simulink model "clearing_faulted_segment_travelling_Wave"  (R2018a)
settings: Solver=ode23t  StartTime=0.0  StopTime=2  MaxStep=1e-3  RelTol=1e-3
values from neighbouring files (symbols this model uses):
  AC_lim = [1.5 -1.5]    [MT_HVDC_initialize.m]
  C_pm = 10.48e-3    (= 0.01048)    [MT_HVDC_initialize.m]
  ccsc_lim = [1.0 -1.0]    [MT_HVDC_initialize.m]
  DC_lim = [1.05 -1.05]    [MT_HVDC_initialize.m]
  f = 50    [MT_HVDC_initialize.m]
  Fc = 50    [MT_HVDC_initialize.m]
  Fn_filter = 1000    [MT_HVDC_initialize.m]
  Ireg_lim_i = [1.5, -1.5]    [MT_HVDC_initialize.m]
  Ireg_lim_r = [1.5, -1.5]    [MT_HVDC_initialize.m]
  Ki_ACreg_i = 260    [MT_HVDC_initialize.m]
  Ki_ccsc = 5    [MT_HVDC_initialize.m]
  Ki_DCreg_r = 150    [MT_HVDC_initialize.m]
  Ki_Ireg_i = 200    [MT_HVDC_initialize.m]
  Ki_Ireg_r = 100    [MT_HVDC_initialize.m]
  Ki_R_inv = 150000    [MT_HVDC_initialize.m]
  Ki_R_rec = 5000    [MT_HVDC_initialize.m]
  Kp_ACreg_i = 2    [MT_HVDC_initialize.m]
  Kp_ccsc = 1    [MT_HVDC_initialize.m]
  Kp_DCreg_r = 8    [MT_HVDC_initialize.m]
  Kp_Ireg_i = 2    [MT_HVDC_initialize.m]
  Kp_Ireg_r = 2    [MT_HVDC_initialize.m]
  Kp_R_inv = 0.001    [MT_HVDC_initialize.m]
  Kp_R_rec = 0.001    [MT_HVDC_initialize.m]
  L1_pu = 0.109    [MT_HVDC_initialize.m]
  L2_pu = 0.0824    [MT_HVDC_initialize.m]
  L_arm = L_arm_pu*Z_base66/w    [MT_HVDC_initialize.m]
  L_arm_pu = 0.15    [MT_HVDC_initialize.m]
  L_int = X_int/w    [MT_HVDC_initialize.m]
  n = 50    [MT_HVDC_initialize.m]
  n2 = 50    [MT_HVDC_initialize.m]
  P_nom = 220e6    (= 220000000)    [MT_HVDC_initialize.m]
  R1_pu = 0.00206    [MT_HVDC_initialize.m]
  R2_pu = 0.00206    [MT_HVDC_initialize.m]
  R_arm = 0.03    [MT_HVDC_initialize.m]
  R_arm_pu = R_arm/Z_base66    [MT_HVDC_initialize.m]
  R_int = sqrt((z_int_400^2)/(1+xr_ratio^2))    [MT_HVDC_initialize.m]
  Rg_T1 = 40    [MT_HVDC_initialize.m]
  S1_nom = P_nom    (= 220000000)    [MT_HVDC_initialize.m]
  S2_nom = P_nom    (= 220000000)    [MT_HVDC_initialize.m]
  T_fault = 1.4    [MT_HVDC_initialize.m]
  Ts_Control = 40e-6    (= 4e-05)    [MT_HVDC_initialize.m]
  Ts_Power = 20e-6    (= 2e-05)    [MT_HVDC_initialize.m]
  V1_prim = V_prim    (= 400000)    [MT_HVDC_initialize.m]
  V1_sec = V_grid    (= 66000)    [MT_HVDC_initialize.m]
  V2_prim = V_grid    (= 66000)    [MT_HVDC_initialize.m]
  V2_sec = 18e3    (= 18000)    [MT_HVDC_initialize.m]
  V_ac_ref = 1.035    [MT_HVDC_initialize.m]
  V_grid = 66e3    (= 66000)    [MT_HVDC_initialize.m]
  V_prim = 400e3    (= 400000)    [MT_HVDC_initialize.m]
  Vc_pm_r = 0*Vdc_nom/n    (= 0)    [MT_HVDC_initialize.m]
  Vdc_nom = 135e3    (= 135000)    [MT_HVDC_initialize.m]
  w = 2*pi*f    (= 314.159265359)    [MT_HVDC_initialize.m]
  z0z1 = 0.8    [MT_HVDC_initialize.m]
  Zeta_filter = 1    [MT_HVDC_initialize.m]
undefined symbols (not defined in the file or in its folder): D1, Delta, DiscIntNeverNeededParam
libraries: powerlib x417, powerlib_meascontrol x130, simulink x84, powerlib_extras x8, simulink_extras x5
(part 7 of 17)

== system clearing_faulted_segment_travelling_Wave/Startup Simulation - Guide ==
  note: Startup guide:
      | 1. Set inititial submodule capacitor voltages to zero in script
      | ********************Sequencer in following order**********************
      | 2. Set time for energize grid filter/transformers T_energize (0.1s)
      | 3. Set time for Circulating Current Suppression T_circ (0.1s)
      | 4. Set time for converter energization T_startup (0.4s)
      | 5. Set time for DC Regulator T_DC_Reg (0.4s)
      | 6. Set time for AC RMS Regulator T_AC_Reg (0.7s)
      | 7. Set time for load switching T_Load_nom (1.0s)

== system clearing_faulted_segment_travelling_Wave/Subsystem ==
  DC regulator TURN ON - (id reference for rectifier) : Step  Time=0.2  SampleTime=0
  Enable AC RMS regulator TURN ON - (id reference for inverter) : Step  Time=0.3  SampleTime=0
  Enable Circulating Current Suppresion : Step  Time=0.1  SampleTime=0
  Switch on load network : Step  Time=0.4  SampleTime=0
  tag scope: T_AC_Reg=global, T_DC_Reg=global, T_Load_nom=global, T_circ_i=global, T_circ_r=global
  wires:
  DC regulator TURN ON - (id reference for rectifier)/1 -> [T_DC_Reg]
  Enable Circulating Current Suppresion/1 -> [T_circ_i], [T_circ_r]
  Enable AC RMS regulator TURN ON - (id reference for inverter)/1 -> [T_AC_Reg]
  Switch on load network/1 -> [T_Load_nom]

== system clearing_faulted_segment_travelling_Wave/Thyristor Static AC BREAKER - Active bypass system ==
  note: This thyristor bypass switch is used for investigation of fault current supply when a fault in the load network occurs, allowing selectivity of the network since the MMC inverter cannot supply this current without taking damage.
  note: To Use: Block inverter and rectifier with logic signal, and enable the thyristor bypass. A control logic might be implemented that automatically detects situation where bypass is needed.
  note: Thyristor Pulse Generation based on PLL syncronization from GRID
  note: Thyristor Bypass System;
      |  Two sync: grid and load
      |    Is the blocking done in both converter at the same time, or rectifier and then inverter?
  Block : Inport
  wt : Inport  Port=2
  Constant : Constant  Value=0
  Constant1 : Constant  Value=pi
  Current Measurement : powerlib/Measurements/Current Measurement  PhasorSimulation=off  OutputType=Complex  PSBequivalent=0
      settings: SourceProductName=Simscape Electrical
  Demux1 : Demux  Outputs=6
  Less Than : RelationalOperator  Operator=<  OutDataTypeStr=boolean  RndMeth=Simplest
  Less Than1 : RelationalOperator  Operator=<  OutDataTypeStr=boolean  RndMeth=Simplest
  Less Than2 : RelationalOperator  Operator=<  OutDataTypeStr=boolean  RndMeth=Simplest
  Logical Operator : Logic  Operator=NOT  AllPortsSameDT=off  OutDataTypeStr=boolean
  Logical Operator1 : Logic  Operator=NOT  AllPortsSameDT=off  OutDataTypeStr=boolean
  Logical Operator2 : Logic  Operator=NOT  AllPortsSameDT=off  OutDataTypeStr=boolean
  Mux : Mux  Inputs=6
  Scope : Scope  NumInputPorts=2
  Switch1 : Switch  Criteria=u2 > Threshold
  Terminator{,1..5} (6 alike) : Terminator
  Thyristor{,1..5} (6 alike) : powerlib/Power Electronics/Thyristor  Ron=0.001  Lon=0  Vf=0.8  IC=0  Rs=500  Cs=250e-9  Measurements=on
      settings: SourceProductName=Simscape Electrical
  Transport Delay : TransportDelay  DelayTime=(1/3)*(1/50)
  Transport Delay1 : TransportDelay  DelayTime=(2/3)*(1/50)
  Voltage Measurement : powerlib/Measurements/Voltage Measurement  PhasorSimulation=off  OutputType=Complex  PSBequivalent=0
      settings: SourceProductName=Simscape Electrical
  a : PMIOPort  Tag=PMCPort  Side=Left
  b : PMIOPort  Tag=PMCPort  Port=2  Side=Left
  c : PMIOPort  Tag=PMCPort  Port=3  Side=Left
  A : PMIOPort  Tag=PMCPort  Port=4  Side=Right
  " B" : PMIOPort  Tag=PMCPort  Port=5  Side=Right
  C : PMIOPort  Tag=PMCPort  Port=6  Side=Right
  wires:
  Block/1 -> Switch1/2
  Voltage Measurement/1 -> Scope/1
  Current Measurement/1 -> Scope/2
  Switch1/1 -> Demux1/1
  Constant/1 -> Switch1/1
  Constant1/1 -> Less Than/2, Less Than1/2, Less Than2/2
  Transport Delay/1 -> Less Than1/1
  Transport Delay1/1 -> Less Than2/1
  Less Than/1 -> Logical Operator/1, Mux/1
  wt/1 -> Transport Delay/1, Transport Delay1/1, Less Than/1
  Logical Operator/1 -> Mux/2
  Logical Operator1/1 -> Mux/4
  Logical Operator2/1 -> Mux/6
  Less Than1/1 -> Logical Operator1/1, Mux/3
  Less Than2/1 -> Logical Operator2/1, Mux/5
  Mux/1 -> Switch1/3
  Demux1/1 -> Thyristor/1
  Demux1/2 -> Thyristor1/1
  Demux1/3 -> Thyristor2/1
  Demux1/4 -> Thyristor3/1
  Demux1/5 -> Thyristor4/1
  Demux1/6 -> Thyristor5/1
  Thyristor/1 -> Terminator/1
  Thyristor2/1 -> Terminator1/1
  Thyristor5/1 -> Terminator2/1
  Thyristor1/1 -> Terminator4/1
  Thyristor3/1 -> Terminator3/1
  Thyristor4/1 -> Terminator5/1
  connections:
  Thyristor1/LConn1 -- Voltage Measurement/LConn2 -- Current Measurement/LConn1 -- Thyristor/RConn1
  Thyristor1/RConn1 -- Thyristor/LConn1 -- Voltage Measurement/LConn1 -- a/RConn1
  b/RConn1 -- Thyristor2/LConn1 -- Thyristor3/RConn1
  Thyristor3/LConn1 -- " B"/RConn1 -- Thyristor2/RConn1
  Thyristor4/LConn1 -- c/RConn1 -- Thyristor5/RConn1
  Thyristor4/RConn1 -- C/RConn1 -- Thyristor5/LConn1
  Current Measurement/RConn1 -- A/RConn1

== system clearing_faulted_segment_travelling_Wave/Controlsystem for Inverter/Dq0 Control ==
  I_ph : Inport
  V_ph : Inport  Port=2
  Circulating current suppression1 : Subsystem  VariantControl=Variant1
  Constant18 : Constant  Value=V_ac_ref
  Constant2 : Constant  Value=1/(Vdc_nom/2*sqrt(3)/sqrt(2)/V_grid)
  Goto8 : Goto  Commented=on  GotoTag=V_diffi_i  TagVisibility=global
  Inncer current loop - Positive and Negative Sequence Control : Subsystem
  "Measurement - dq0 positiveand negative sequence, - and zero sequence in alphabetta - Rectifier" : Subsystem
  Outer loop - AC RMS controller1 : Subsystem
  PWM Signal Generator - Inverter1 : Subsystem
  Rate Transition1 : RateTransition  OutPortSampleTime=Ts_Power
  Reactive power Set-point : Subsystem
  Zero Sequence Controller : Subsystem
  Control Signal1 : Outport
  tag scope: m_i_pn=global
  wires:
  "Measurement - dq0 positiveand negative sequence, - and zero sequence in alphabetta - Rectifier"/3(wt) -> Inncer current loop - Positive and Negative Sequence Control/5(wt)
  [T_AC_Reg] -> Outer loop - AC RMS controller1/3(Enable)
  [T_iq_reg_i] -> Reactive power Set-point/Enable, Reactive power Set-point/1(T_Qreg_on)
  [PQ_i] -> Reactive power Set-point/2(Q_ref)
  [I_arm_i] -> Circulating current suppression1/2(I_arm)
  [T_zero] -> Zero Sequence Controller/Enable, Zero Sequence Controller/3(Enable)
  [T_Block_i] -> PWM Signal Generator - Inverter1/2(Block)
  Zero Sequence Controller/1(V_zero_ref) -> Inncer current loop - Positive and Negative Sequence Control/7(V_ref_zero)
  Constant2/1 -> Inncer current loop - Positive and Negative Sequence Control/6(Vdc_pu)
  Inncer current loop - Positive and Negative Sequence Control/1(m_ref) -> [m_i_pn], Rate Transition1/1
  "Measurement - dq0 positiveand negative sequence, - and zero sequence in alphabetta - Rectifier"/4(V_zero) -> Zero Sequence Controller/1(V0_meas)
  PWM Signal Generator - Inverter1/1(g) -> Control Signal1/1
  Circulating current suppression1/1(V_diffi) -> Inncer current loop - Positive and Negative Sequence Control/8(V_diffi), Goto8/1
  Rate Transition1/1 -> PWM Signal Generator - Inverter1/1(U_ref)
  [T_circ_i] -> Circulating current suppression1/Enable, Circulating current suppression1/1(Enable)
  "Measurement - dq0 positiveand negative sequence, - and zero sequence in alphabetta - Rectifier"/5(I_zero) -> Zero Sequence Controller/2(I0_meas)
  Constant18/1 -> Outer loop - AC RMS controller1/1(Vac_ref)
  Outer loop - AC RMS controller1/1(Id_ref) -> Inncer current loop - Positive and Negative Sequence Control/1(id_pos_ref)
  Reactive power Set-point/1(Iq_ref) -> Inncer current loop - Positive and Negative Sequence Control/2(iq_pos_ref)
  "Measurement - dq0 positiveand negative sequence, - and zero sequence in alphabetta - Rectifier"/2(Vdq) -> Reactive power Set-point/3(Vdq+), Outer loop - AC RMS controller1/2(vdq+), Inncer current loop - Positive and Negative Sequence Control/4(Vdq+)
  "Measurement - dq0 positiveand negative sequence, - and zero sequence in alphabetta - Rectifier"/1(Idq) -> Inncer current loop - Positive and Negative Sequence Control/3(Idq+)
  I_ph/1 -> "Measurement - dq0 positiveand negative sequence, - and zero sequence in alphabetta - Rectifier"/2(I_ph)
  V_ph/1 -> "Measurement - dq0 positiveand negative sequence, - and zero sequence in alphabetta - Rectifier"/1(V_ph)

== system clearing_faulted_segment_travelling_Wave/Controlsystem for Inverter/Dq0 control with Dual Synchronous Reference Frame (DSRF) ==
  I_ph : Inport
  V_ph : Inport  Port=2
  Circulating current suppression1 : Subsystem  VariantControl=Variant1
  Constant : Constant  Value=V_ac_ref
  Constant2 : Constant  Value=1/(Vdc_nom/2*sqrt(3)/sqrt(2)/V_grid)
  Goto8 : Goto  Commented=on  GotoTag=V_diffi_i  TagVisibility=global
  Inncer current loop - Positive and Negative Sequence Control : Subsystem
  "Measurement - dq0 positiveand negative sequence, - and zero sequence in alphabetta2" : Subsystem
  Outer loop - AC RMS controller1 : Subsystem
  PWM Signal Generator - Inverter1 : Subsystem
  Rate Transition1 : RateTransition  OutPortSampleTime=Ts_Power
  Reactive power Set-point : Subsystem
  Zero Sequence Controller2 : Subsystem
  Control Signal1 : Outport
  tag scope: m_i_pn=global
  wires:
  "Measurement - dq0 positiveand negative sequence, - and zero sequence in alphabetta2"/3(Vdq+) -> Outer loop - AC RMS controller1/2(vdq+), Inncer current loop - Positive and Negative Sequence Control/5(Vdq+), Reactive power Set-point/3(Vdq+)
  "Measurement - dq0 positiveand negative sequence, - and zero sequence in alphabetta2"/4(Vdq-) -> Inncer current loop - Positive and Negative Sequence Control/6(Vdq-)
  [T_AC_Reg] -> Outer loop - AC RMS controller1/3(Enable)
  [T_iq_reg_i] -> Reactive power Set-point/Enable, Reactive power Set-point/1(T_Qreg_on)
  V_ph/1 -> "Measurement - dq0 positiveand negative sequence, - and zero sequence in alphabetta2"/2(V_ph)
  [PQ_i] -> Reactive power Set-point/2(Q_ref)
  I_ph/1 -> "Measurement - dq0 positiveand negative sequence, - and zero sequence in alphabetta2"/1(I_ph)
  Reactive power Set-point/1(Iq_ref) -> Inncer current loop - Positive and Negative Sequence Control/2(iq_pos_ref)
  "Measurement - dq0 positiveand negative sequence, - and zero sequence in alphabetta2"/2(Idq-) -> Inncer current loop - Positive and Negative Sequence Control/4(Idq-)
  [I_arm_i] -> Circulating current suppression1/2(I_arm)
  "Measurement - dq0 positiveand negative sequence, - and zero sequence in alphabetta2"/1(Idq+) -> Inncer current loop - Positive and Negative Sequence Control/3(Idq+)
  [T_zero] -> Zero Sequence Controller2/Enable, Zero Sequence Controller2/3(Enable)
  [T_Block_i] -> PWM Signal Generator - Inverter1/2(Block)
  Zero Sequence Controller2/1(V_zero_ref) -> Inncer current loop - Positive and Negative Sequence Control/9(V_ref_zero)
  Constant2/1 -> Inncer current loop - Positive and Negative Sequence Control/8(Vdc_pu)
  Inncer current loop - Positive and Negative Sequence Control/1(m_ref) -> [m_i_pn], Rate Transition1/1
  "Measurement - dq0 positiveand negative sequence, - and zero sequence in alphabetta2"/5(wt) -> Inncer current loop - Positive and Negative Sequence Control/7(wt)
  "Measurement - dq0 positiveand negative sequence, - and zero sequence in alphabetta2"/6(V_zero) -> Zero Sequence Controller2/1(V0_meas)
  PWM Signal Generator - Inverter1/1(g) -> Control Signal1/1
  Circulating current suppression1/1(V_diffi) -> Inncer current loop - Positive and Negative Sequence Control/10(V_diffi), Goto8/1
  Rate Transition1/1 -> PWM Signal Generator - Inverter1/1(U_ref)
  [T_circ_i] -> Circulating current suppression1/Enable, Circulating current suppression1/1(Enable)
  "Measurement - dq0 positiveand negative sequence, - and zero sequence in alphabetta2"/7(I_zero) -> Zero Sequence Controller2/2(I0_meas)
  Outer loop - AC RMS controller1/1(Id_ref) -> Inncer current loop - Positive and Negative Sequence Control/1(id_pos_ref)
  Constant/1 -> Outer loop - AC RMS controller1/1(Vac_ref)

== system clearing_faulted_segment_travelling_Wave/Controlsystem for rectifier/Dq0 Control ==
  I_ph : Inport
  V_ph : Inport  Port=2
  V_dc : Inport  Port=3
  AC Voltage Controller : Subsystem
  Circulating current suppression : Subsystem  VariantControl=Variant1
  Constant1 : Constant  Value=1/(Vdc_nom/2*sqrt(3)/sqrt(2)/V_grid)
  Constant2 : Constant  Value=Vdc_nom
  Constant6 : Constant  Value=V_grid
  DC voltage control - Outer loop : Subsystem
  Inncer current loop - Positive and Negative Sequence Control : Subsystem
  "Measurement - dq0 positiveand negative sequence, - and zero sequence in alphabetta - Rectifier" : Subsystem
  PWM Signal Generator - Rectifier : Subsystem
  Rate Transition1 : RateTransition  OutPortSampleTime=Ts_Power
  Step : Step  Time=(T_fault+0.15)  Before=[DC_lim(1) DC_lim(2)]  After=[DC_lim(1) DC_lim(2)]  SampleTime=0
  Zero Sequence Controller2 : Subsystem
  Control Signal : Outport
  wt : Outport  Port=2
  tag scope: V_diffi_r=global, m_r_pn=global
  wires:
  Circulating current suppression/1(V_diffi) -> Inncer current loop - Positive and Negative Sequence Control/8(V_diffi), [V_diffi_r]
  [T_circ_r] -> Circulating current suppression/1(Enable), Circulating current suppression/Enable
  [I_arm_r] -> Circulating current suppression/2(I_arm)
  AC Voltage Controller/1(Iq_ref) -> Inncer current loop - Positive and Negative Sequence Control/2(iq_pos_ref)
  [T_iq_reg_r] -> AC Voltage Controller/Enable, AC Voltage Controller/1("Enable ")
  V_ph/1 -> AC Voltage Controller/3(V_ac), "Measurement - dq0 positiveand negative sequence, - and zero sequence in alphabetta - Rectifier"/1(V_ph)
  Constant6/1 -> AC Voltage Controller/2(V_ac_ref)
  [T_zero] -> Zero Sequence Controller2/3(Enable), Zero Sequence Controller2/Enable
  Step/1 -> DC voltage control - Outer loop/4(DC_limit)
  Constant1/1 -> Inncer current loop - Positive and Negative Sequence Control/6(Vdc_pu)
  Zero Sequence Controller2/1(V_zero_ref) -> Inncer current loop - Positive and Negative Sequence Control/7(V_ref_zero)
  "Measurement - dq0 positiveand negative sequence, - and zero sequence in alphabetta - Rectifier"/2(Vdq) -> Inncer current loop - Positive and Negative Sequence Control/4(Vdq+)
  Inncer current loop - Positive and Negative Sequence Control/1(m_ref) -> [m_r_pn], Rate Transition1/1
  "Measurement - dq0 positiveand negative sequence, - and zero sequence in alphabetta - Rectifier"/5(I_zero) -> Zero Sequence Controller2/2(I0_meas)
  DC voltage control - Outer loop/1(Id_ref) -> Inncer current loop - Positive and Negative Sequence Control/1(id_pos_ref)
  [T_DC_Reg] -> DC voltage control - Outer loop/3(Enable)
  "Measurement - dq0 positiveand negative sequence, - and zero sequence in alphabetta - Rectifier"/1(Idq) -> Inncer current loop - Positive and Negative Sequence Control/3(Idq+)
  "Measurement - dq0 positiveand negative sequence, - and zero sequence in alphabetta - Rectifier"/3(wt) -> wt/1, Inncer current loop - Positive and Negative Sequence Control/5(wt)
  "Measurement - dq0 positiveand negative sequence, - and zero sequence in alphabetta - Rectifier"/4(V_zero) -> Zero Sequence Controller2/1(V0_meas)
  [T_Block_r] -> PWM Signal Generator - Rectifier/2(Block)
  V_dc/1 -> DC voltage control - Outer loop/1(V_dc_meas)
  I_ph/1 -> "Measurement - dq0 positiveand negative sequence, - and zero sequence in alphabetta - Rectifier"/2(I_ph)
  PWM Signal Generator - Rectifier/1(g) -> Control Signal/1
  Rate Transition1/1 -> PWM Signal Generator - Rectifier/1(U_ref)
  Constant2/1 -> DC voltage control - Outer loop/2(V_dc_ref)

== system clearing_faulted_segment_travelling_Wave/Controlsystem for rectifier/Dq0 Control with Dual Synchronous Reference Frame (DSRF) ==
  I_ph : Inport
  V_ph : Inport  Port=2
  V_dc : Inport  Port=3
  AC Voltage Controller : Subsystem
  Circulating current suppression : Subsystem  VariantControl=Variant1
  Constant1 : Constant  Value=1/(Vdc_nom/2*sqrt(3)/sqrt(2)/V_grid)
  Constant2 : Constant  Value=Vdc_nom
  Constant6 : Constant
  DC voltage control - Outer loop : Subsystem
  Inner Current loop - Positive and Negative Sequence Control - Rectifier : Subsystem
  "Measurement - dq0 positiveand negative sequence, - and zero sequence in alphabetta - Rectifier" : Subsystem
  PWM Signal Generator - Rectifier : Subsystem
  Rate Transition1 : RateTransition  OutPortSampleTime=Ts_Power
  Step : Step  Time=(T_fault+0.15)  Before=[DC_lim(1) DC_lim(2)]  After=[DC_lim(1) DC_lim(2)]  SampleTime=0
  Zero Sequence Controller2 : Subsystem
  Control Signal : Outport
  wt : Outport  Port=2
  tag scope: V_diffi_r=global, m_r_pn=global
  wires:
  Rate Transition1/1 -> PWM Signal Generator - Rectifier/1(U_ref)
  PWM Signal Generator - Rectifier/1(g) -> Control Signal/1
  I_ph/1 -> "Measurement - dq0 positiveand negative sequence, - and zero sequence in alphabetta - Rectifier"/2(I_ph)
  V_dc/1 -> DC voltage control - Outer loop/1(V_dc_meas)
  [T_Block_r] -> PWM Signal Generator - Rectifier/2(Block)
  "Measurement - dq0 positiveand negative sequence, - and zero sequence in alphabetta - Rectifier"/6(V_zero) -> Zero Sequence Controller2/1(V0_meas)
  "Measurement - dq0 positiveand negative sequence, - and zero sequence in alphabetta - Rectifier"/5(wt) -> wt/1, Inner Current loop - Positive and Negative Sequence Control - Rectifier/7(wt)
  "Measurement - dq0 positiveand negative sequence, - and zero sequence in alphabetta - Rectifier"/1(Idq+) -> Inner Current loop - Positive and Negative Sequence Control - Rectifier/3(Idq+)
  [T_DC_Reg] -> DC voltage control - Outer loop/3(Enable)
  "Measurement - dq0 positiveand negative sequence, - and zero sequence in alphabetta - Rectifier"/7(I_zero) -> Zero Sequence Controller2/2(I0_meas)
  Inner Current loop - Positive and Negative Sequence Control - Rectifier/1(m_ref) -> [m_r_pn], Rate Transition1/1
  "Measurement - dq0 positiveand negative sequence, - and zero sequence in alphabetta - Rectifier"/3(Vdq+) -> AC Voltage Controller/3(Vdq+), Inner Current loop - Positive and Negative Sequence Control - Rectifier/5(Vdq+)
  "Measurement - dq0 positiveand negative sequence, - and zero sequence in alphabetta - Rectifier"/4(Vdq-) -> Inner Current loop - Positive and Negative Sequence Control - Rectifier/6(Vdq-)
  "Measurement - dq0 positiveand negative sequence, - and zero sequence in alphabetta - Rectifier"/2(Idq-) -> Inner Current loop - Positive and Negative Sequence Control - Rectifier/4(Idq-)
  Zero Sequence Controller2/1(V_zero_ref) -> Inner Current loop - Positive and Negative Sequence Control - Rectifier/9(V_ref_zero)
  Constant1/1 -> Inner Current loop - Positive and Negative Sequence Control - Rectifier/8(Vdc_pu)
  Step/1 -> DC voltage control - Outer loop/4(DC_limit)
  [T_zero] -> Zero Sequence Controller2/Enable, Zero Sequence Controller2/3(Enable)
  Constant6/1 -> AC Voltage Controller/2(V_ac_ref)
  V_ph/1 -> "Measurement - dq0 positiveand negative sequence, - and zero sequence in alphabetta - Rectifier"/1(V_ph)
  [T_iq_reg_r] -> AC Voltage Controller/1("Enable "), AC Voltage Controller/Enable
  AC Voltage Controller/1(Iq_ref) -> Inner Current loop - Positive and Negative Sequence Control - Rectifier/2(iq_pos_ref)
  [I_arm_r] -> Circulating current suppression/2(I_arm)
  [T_circ_r] -> Circulating current suppression/Enable, Circulating current suppression/1(Enable)
  Circulating current suppression/1(V_diffi) -> Inner Current loop - Positive and Negative Sequence Control - Rectifier/10(V_diffi), [V_diffi_r]
  Constant2/1 -> DC voltage control - Outer loop/2(V_dc_ref)
  DC voltage control - Outer loop/1(Id_ref) -> Inner Current loop - Positive and Negative Sequence Control - Rectifier/1(id_pos_ref)

== system clearing_faulted_segment_travelling_Wave/Controlsystem for rectifier1/Dq0 Control ==
  I_ph : Inport
  V_ph : Inport  Port=2
  V_dc : Inport  Port=3
  AC Voltage Controller : Subsystem
  Circulating current suppression : Subsystem  VariantControl=Variant1
  Constant1 : Constant  Value=1/(Vdc_nom/2*sqrt(3)/sqrt(2)/V_grid)
  Constant2 : Constant  Value=Vdc_nom
  Constant6 : Constant  Value=V_grid
  DC voltage control - Outer loop : Subsystem
  Inncer current loop - Positive and Negative Sequence Control : Subsystem
  "Measurement - dq0 positiveand negative sequence, - and zero sequence in alphabetta - Rectifier" : Subsystem
  PWM Signal Generator - Rectifier : Subsystem
  Rate Transition1 : RateTransition  OutPortSampleTime=Ts_Power
  Step : Step  Time=(T_fault+0.15)  Before=[DC_lim(1) DC_lim(2)]  After=[DC_lim(1) DC_lim(2)]  SampleTime=0
  Zero Sequence Controller2 : Subsystem
  Control Signal : Outport
  wt : Outport  Port=2
  tag scope: V_diffi_r2=global, m_r_pn2=global
  wires:
  Circulating current suppression/1(V_diffi) -> Inncer current loop - Positive and Negative Sequence Control/8(V_diffi), [V_diffi_r2]
  [T_circ_r] -> Circulating current suppression/1(Enable), Circulating current suppression/Enable
  [I_arm_r2] -> Circulating current suppression/2(I_arm)
  AC Voltage Controller/1(Iq_ref) -> Inncer current loop - Positive and Negative Sequence Control/2(iq_pos_ref)
  [T_iq_reg_r] -> AC Voltage Controller/Enable, AC Voltage Controller/1("Enable ")
  V_ph/1 -> AC Voltage Controller/3(V_ac), "Measurement - dq0 positiveand negative sequence, - and zero sequence in alphabetta - Rectifier"/1(V_ph)
  Constant6/1 -> AC Voltage Controller/2(V_ac_ref)
  [T_zero] -> Zero Sequence Controller2/3(Enable), Zero Sequence Controller2/Enable
  Step/1 -> DC voltage control - Outer loop/4(DC_limit)
  Constant1/1 -> Inncer current loop - Positive and Negative Sequence Control/6(Vdc_pu)
  Zero Sequence Controller2/1(V_zero_ref) -> Inncer current loop - Positive and Negative Sequence Control/7(V_ref_zero)
  "Measurement - dq0 positiveand negative sequence, - and zero sequence in alphabetta - Rectifier"/2(Vdq) -> Inncer current loop - Positive and Negative Sequence Control/4(Vdq+)
  Inncer current loop - Positive and Negative Sequence Control/1(m_ref) -> [m_r_pn2], Rate Transition1/1
  "Measurement - dq0 positiveand negative sequence, - and zero sequence in alphabetta - Rectifier"/5(I_zero) -> Zero Sequence Controller2/2(I0_meas)
  DC voltage control - Outer loop/1(Id_ref) -> Inncer current loop - Positive and Negative Sequence Control/1(id_pos_ref)
  [T_DC_Reg] -> DC voltage control - Outer loop/3(Enable)
  "Measurement - dq0 positiveand negative sequence, - and zero sequence in alphabetta - Rectifier"/1(Idq) -> Inncer current loop - Positive and Negative Sequence Control/3(Idq+)
  "Measurement - dq0 positiveand negative sequence, - and zero sequence in alphabetta - Rectifier"/3(wt) -> wt/1, Inncer current loop - Positive and Negative Sequence Control/5(wt)
  "Measurement - dq0 positiveand negative sequence, - and zero sequence in alphabetta - Rectifier"/4(V_zero) -> Zero Sequence Controller2/1(V0_meas)
  [T_Block_r] -> PWM Signal Generator - Rectifier/2(Block)
  V_dc/1 -> DC voltage control - Outer loop/1(V_dc_meas)
  I_ph/1 -> "Measurement - dq0 positiveand negative sequence, - and zero sequence in alphabetta - Rectifier"/2(I_ph)
  PWM Signal Generator - Rectifier/1(g) -> Control Signal/1
  Rate Transition1/1 -> PWM Signal Generator - Rectifier/1(U_ref)
  Constant2/1 -> DC voltage control - Outer loop/2(V_dc_ref)

== system clearing_faulted_segment_travelling_Wave/Controlsystem for rectifier1/Dq0 Control with Dual Synchronous Reference Frame (DSRF) ==
  I_ph : Inport
  V_ph : Inport  Port=2
  V_dc : Inport  Port=3
  AC Voltage Controller : Subsystem
  Circulating current suppression : Subsystem  VariantControl=Variant1
  Constant1 : Constant  Value=1/(Vdc_nom/2*sqrt(3)/sqrt(2)/V_grid)
  Constant2 : Constant  Value=Vdc_nom
  Constant6 : Constant
  DC voltage control - Outer loop : Subsystem
  Inner Current loop - Positive and Negative Sequence Control - Rectifier : Subsystem
  "Measurement - dq0 positiveand negative sequence, - and zero sequence in alphabetta - Rectifier" : Subsystem
  PWM Signal Generator - Rectifier : Subsystem
  Rate Transition1 : RateTransition  OutPortSampleTime=Ts_Power
  Step : Step  Time=(T_fault+0.15)  Before=[DC_lim(1) DC_lim(2)]  After=[DC_lim(1) DC_lim(2)]  SampleTime=0
  Zero Sequence Controller2 : Subsystem
  Control Signal : Outport
  wt : Outport  Port=2
  tag scope: V_diffi_r=global, m_r_pn=global
  wires:
  Rate Transition1/1 -> PWM Signal Generator - Rectifier/1(U_ref)
  PWM Signal Generator - Rectifier/1(g) -> Control Signal/1
  I_ph/1 -> "Measurement - dq0 positiveand negative sequence, - and zero sequence in alphabetta - Rectifier"/2(I_ph)
  V_dc/1 -> DC voltage control - Outer loop/1(V_dc_meas)
  [T_Block_r] -> PWM Signal Generator - Rectifier/2(Block)
  "Measurement - dq0 positiveand negative sequence, - and zero sequence in alphabetta - Rectifier"/6(V_zero) -> Zero Sequence Controller2/1(V0_meas)
  "Measurement - dq0 positiveand negative sequence, - and zero sequence in alphabetta - Rectifier"/5(wt) -> wt/1, Inner Current loop - Positive and Negative Sequence Control - Rectifier/7(wt)
  "Measurement - dq0 positiveand negative sequence, - and zero sequence in alphabetta - Rectifier"/1(Idq+) -> Inner Current loop - Positive and Negative Sequence Control - Rectifier/3(Idq+)
  [T_DC_Reg] -> DC voltage control - Outer loop/3(Enable)
  "Measurement - dq0 positiveand negative sequence, - and zero sequence in alphabetta - Rectifier"/7(I_zero) -> Zero Sequence Controller2/2(I0_meas)
  Inner Current loop - Positive and Negative Sequence Control - Rectifier/1(m_ref) -> [m_r_pn], Rate Transition1/1
  "Measurement - dq0 positiveand negative sequence, - and zero sequence in alphabetta - Rectifier"/3(Vdq+) -> AC Voltage Controller/3(Vdq+), Inner Current loop - Positive and Negative Sequence Control - Rectifier/5(Vdq+)
  "Measurement - dq0 positiveand negative sequence, - and zero sequence in alphabetta - Rectifier"/4(Vdq-) -> Inner Current loop - Positive and Negative Sequence Control - Rectifier/6(Vdq-)
  "Measurement - dq0 positiveand negative sequence, - and zero sequence in alphabetta - Rectifier"/2(Idq-) -> Inner Current loop - Positive and Negative Sequence Control - Rectifier/4(Idq-)
  Zero Sequence Controller2/1(V_zero_ref) -> Inner Current loop - Positive and Negative Sequence Control - Rectifier/9(V_ref_zero)
  Constant1/1 -> Inner Current loop - Positive and Negative Sequence Control - Rectifier/8(Vdc_pu)
  Step/1 -> DC voltage control - Outer loop/4(DC_limit)
  [T_zero] -> Zero Sequence Controller2/Enable, Zero Sequence Controller2/3(Enable)
  Constant6/1 -> AC Voltage Controller/2(V_ac_ref)
  V_ph/1 -> "Measurement - dq0 positiveand negative sequence, - and zero sequence in alphabetta - Rectifier"/1(V_ph)
  [T_iq_reg_r] -> AC Voltage Controller/1("Enable "), AC Voltage Controller/Enable
  AC Voltage Controller/1(Iq_ref) -> Inner Current loop - Positive and Negative Sequence Control - Rectifier/2(iq_pos_ref)
  [I_arm_r] -> Circulating current suppression/2(I_arm)
  [T_circ_r] -> Circulating current suppression/Enable, Circulating current suppression/1(Enable)
  Circulating current suppression/1(V_diffi) -> Inner Current loop - Positive and Negative Sequence Control - Rectifier/10(V_diffi), [V_diffi_r]
  Constant2/1 -> DC voltage control - Outer loop/2(V_dc_ref)
  DC voltage control - Outer loop/1(Id_ref) -> Inner Current loop - Positive and Negative Sequence Control - Rectifier/1(id_pos_ref)

== system clearing_faulted_segment_travelling_Wave/Controlsystem for rectifier2/Dq0 Control ==
  I_ph : Inport
  V_ph : Inport  Port=2
  V_dc : Inport  Port=3
  AC Voltage Controller : Subsystem
  Circulating current suppression : Subsystem  VariantControl=Variant1
  Constant1 : Constant  Value=1/(Vdc_nom/2*sqrt(3)/sqrt(2)/V_grid)
  Constant2 : Constant  Value=Vdc_nom
  Constant6 : Constant  Value=V_grid
  DC voltage control - Outer loop : Subsystem
  Inncer current loop - Positive and Negative Sequence Control : Subsystem
  "Measurement - dq0 positiveand negative sequence, - and zero sequence in alphabetta - Rectifier" : Subsystem
  PWM Signal Generator - Rectifier : Subsystem
  Rate Transition1 : RateTransition  OutPortSampleTime=Ts_Power
  Step : Step  Time=(T_fault+0.15)  Before=[DC_lim(1) DC_lim(2)]  After=[DC_lim(1) DC_lim(2)]  SampleTime=0
  Zero Sequence Controller2 : Subsystem
  Control Signal : Outport
  wt : Outport  Port=2
  tag scope: V_diffi_r3=global, m_r_pn3=global
  wires:
  Circulating current suppression/1(V_diffi) -> Inncer current loop - Positive and Negative Sequence Control/8(V_diffi), [V_diffi_r3]
  [T_circ_r] -> Circulating current suppression/1(Enable), Circulating current suppression/Enable
  [I_arm_r2] -> Circulating current suppression/2(I_arm)
  AC Voltage Controller/1(Iq_ref) -> Inncer current loop - Positive and Negative Sequence Control/2(iq_pos_ref)
  [T_iq_reg_r] -> AC Voltage Controller/Enable, AC Voltage Controller/1("Enable ")
  V_ph/1 -> AC Voltage Controller/3(V_ac), "Measurement - dq0 positiveand negative sequence, - and zero sequence in alphabetta - Rectifier"/1(V_ph)
  Constant6/1 -> AC Voltage Controller/2(V_ac_ref)
  [T_zero] -> Zero Sequence Controller2/3(Enable), Zero Sequence Controller2/Enable
  Step/1 -> DC voltage control - Outer loop/4(DC_limit)
  Constant1/1 -> Inncer current loop - Positive and Negative Sequence Control/6(Vdc_pu)
  Zero Sequence Controller2/1(V_zero_ref) -> Inncer current loop - Positive and Negative Sequence Control/7(V_ref_zero)
  "Measurement - dq0 positiveand negative sequence, - and zero sequence in alphabetta - Rectifier"/2(Vdq) -> Inncer current loop - Positive and Negative Sequence Control/4(Vdq+)
  Inncer current loop - Positive and Negative Sequence Control/1(m_ref) -> [m_r_pn3], Rate Transition1/1
  "Measurement - dq0 positiveand negative sequence, - and zero sequence in alphabetta - Rectifier"/5(I_zero) -> Zero Sequence Controller2/2(I0_meas)
  DC voltage control - Outer loop/1(Id_ref) -> Inncer current loop - Positive and Negative Sequence Control/1(id_pos_ref)
  [T_DC_Reg] -> DC voltage control - Outer loop/3(Enable)
  "Measurement - dq0 positiveand negative sequence, - and zero sequence in alphabetta - Rectifier"/1(Idq) -> Inncer current loop - Positive and Negative Sequence Control/3(Idq+)
  "Measurement - dq0 positiveand negative sequence, - and zero sequence in alphabetta - Rectifier"/3(wt) -> wt/1, Inncer current loop - Positive and Negative Sequence Control/5(wt)
  "Measurement - dq0 positiveand negative sequence, - and zero sequence in alphabetta - Rectifier"/4(V_zero) -> Zero Sequence Controller2/1(V0_meas)
  [T_Block_r] -> PWM Signal Generator - Rectifier/2(Block)
  V_dc/1 -> DC voltage control - Outer loop/1(V_dc_meas)
  I_ph/1 -> "Measurement - dq0 positiveand negative sequence, - and zero sequence in alphabetta - Rectifier"/2(I_ph)
  PWM Signal Generator - Rectifier/1(g) -> Control Signal/1
  Rate Transition1/1 -> PWM Signal Generator - Rectifier/1(U_ref)
  Constant2/1 -> DC voltage control - Outer loop/2(V_dc_ref)

== system clearing_faulted_segment_travelling_Wave/Controlsystem for rectifier2/Dq0 Control with Dual Synchronous Reference Frame (DSRF) ==
  I_ph : Inport
  V_ph : Inport  Port=2
  V_dc : Inport  Port=3
  AC Voltage Controller : Subsystem
  Circulating current suppression : Subsystem  VariantControl=Variant1
  Constant1 : Constant  Value=1/(Vdc_nom/2*sqrt(3)/sqrt(2)/V_grid)
  Constant2 : Constant  Value=Vdc_nom
  Constant6 : Constant
  DC voltage control - Outer loop : Subsystem
  Inner Current loop - Positive and Negative Sequence Control - Rectifier : Subsystem
  "Measurement - dq0 positiveand negative sequence, - and zero sequence in alphabetta - Rectifier" : Subsystem
  PWM Signal Generator - Rectifier : Subsystem
  Rate Transition1 : RateTransition  OutPortSampleTime=Ts_Power
  Step : Step  Time=(T_fault+0.15)  Before=[DC_lim(1) DC_lim(2)]  After=[DC_lim(1) DC_lim(2)]  SampleTime=0
  Zero Sequence Controller2 : Subsystem
  Control Signal : Outport
  wt : Outport  Port=2
  tag scope: V_diffi_r=global, m_r_pn=global
  wires:
  Rate Transition1/1 -> PWM Signal Generator - Rectifier/1(U_ref)
  PWM Signal Generator - Rectifier/1(g) -> Control Signal/1
  I_ph/1 -> "Measurement - dq0 positiveand negative sequence, - and zero sequence in alphabetta - Rectifier"/2(I_ph)
  V_dc/1 -> DC voltage control - Outer loop/1(V_dc_meas)
  [T_Block_r] -> PWM Signal Generator - Rectifier/2(Block)
  "Measurement - dq0 positiveand negative sequence, - and zero sequence in alphabetta - Rectifier"/6(V_zero) -> Zero Sequence Controller2/1(V0_meas)
  "Measurement - dq0 positiveand negative sequence, - and zero sequence in alphabetta - Rectifier"/5(wt) -> wt/1, Inner Current loop - Positive and Negative Sequence Control - Rectifier/7(wt)
  "Measurement - dq0 positiveand negative sequence, - and zero sequence in alphabetta - Rectifier"/1(Idq+) -> Inner Current loop - Positive and Negative Sequence Control - Rectifier/3(Idq+)
  [T_DC_Reg] -> DC voltage control - Outer loop/3(Enable)
  "Measurement - dq0 positiveand negative sequence, - and zero sequence in alphabetta - Rectifier"/7(I_zero) -> Zero Sequence Controller2/2(I0_meas)
  Inner Current loop - Positive and Negative Sequence Control - Rectifier/1(m_ref) -> [m_r_pn], Rate Transition1/1
  "Measurement - dq0 positiveand negative sequence, - and zero sequence in alphabetta - Rectifier"/3(Vdq+) -> AC Voltage Controller/3(Vdq+), Inner Current loop - Positive and Negative Sequence Control - Rectifier/5(Vdq+)
  "Measurement - dq0 positiveand negative sequence, - and zero sequence in alphabetta - Rectifier"/4(Vdq-) -> Inner Current loop - Positive and Negative Sequence Control - Rectifier/6(Vdq-)
  "Measurement - dq0 positiveand negative sequence, - and zero sequence in alphabetta - Rectifier"/2(Idq-) -> Inner Current loop - Positive and Negative Sequence Control - Rectifier/4(Idq-)
  Zero Sequence Controller2/1(V_zero_ref) -> Inner Current loop - Positive and Negative Sequence Control - Rectifier/9(V_ref_zero)
  Constant1/1 -> Inner Current loop - Positive and Negative Sequence Control - Rectifier/8(Vdc_pu)
  Step/1 -> DC voltage control - Outer loop/4(DC_limit)
  [T_zero] -> Zero Sequence Controller2/Enable, Zero Sequence Controller2/3(Enable)
  Constant6/1 -> AC Voltage Controller/2(V_ac_ref)
  V_ph/1 -> "Measurement - dq0 positiveand negative sequence, - and zero sequence in alphabetta - Rectifier"/1(V_ph)
  [T_iq_reg_r] -> AC Voltage Controller/1("Enable "), AC Voltage Controller/Enable
  AC Voltage Controller/1(Iq_ref) -> Inner Current loop - Positive and Negative Sequence Control - Rectifier/2(iq_pos_ref)
  [I_arm_r] -> Circulating current suppression/2(I_arm)
  [T_circ_r] -> Circulating current suppression/Enable, Circulating current suppression/1(Enable)
  Circulating current suppression/1(V_diffi) -> Inner Current loop - Positive and Negative Sequence Control - Rectifier/10(V_diffi), [V_diffi_r]
  Constant2/1 -> DC voltage control - Outer loop/2(V_dc_ref)
  DC voltage control - Outer loop/1(Id_ref) -> Inner Current loop - Positive and Negative Sequence Control - Rectifier/1(id_pos_ref)

== system clearing_faulted_segment_travelling_Wave/MMC Converter1/Half-Bridge MMC Ap ==
  g : Inport
  HalfBridgeMMC_Agt_Discrete : Subsystem  mask{n=n, C=C, Vc_Initial=Vc_Initial, Ron_Diode=1e-3, Rs_Diode=1e6, Cs_Diode=inf, Vf_Diode=0}
      mask prompts: n "Number of bridges:"; C "Capacitor value (F):"; Vc_Initial "Initial capacitor voltage (V):"; Ron_Diode "Diode on-state resistance (Ohms)"; Rs_Diode "Diode snubber resistance (Ohms)"; Cs_Diode "Diode snubber capacitance (F)"; Vf_Diode "Diode forward voltage (V)"
  1 : PMIOPort  Side=Left
  2 : PMIOPort  Port=2  Side=Left
  Vc : Outport
  wires:
  HalfBridgeMMC_Agt_Discrete/1(Vc) -> Vc/1
  g/1 -> HalfBridgeMMC_Agt_Discrete/1(N)
  connections:
  1/RConn1 -- HalfBridgeMMC_Agt_Discrete/LConn1
  2/RConn1 -- HalfBridgeMMC_Agt_Discrete/LConn2

== system clearing_faulted_segment_travelling_Wave/MMC Converter1/Half-Bridge MMC Ap1 ==
  g : Inport
  HalfBridgeMMC_Agt_Discrete : Subsystem  mask{n=n, C=C, Vc_Initial=Vc_Initial, Ron_Diode=1e-3, Rs_Diode=1e6, Cs_Diode=inf, Vf_Diode=0}
      mask prompts: n "Number of bridges:"; C "Capacitor value (F):"; Vc_Initial "Initial capacitor voltage (V):"; Ron_Diode "Diode on-state resistance (Ohms)"; Rs_Diode "Diode snubber resistance (Ohms)"; Cs_Diode "Diode snubber capacitance (F)"; Vf_Diode "Diode forward voltage (V)"
  1 : PMIOPort  Side=Left
  2 : PMIOPort  Port=2  Side=Left
  Vc : Outport
  wires:
  HalfBridgeMMC_Agt_Discrete/1(Vc) -> Vc/1
  g/1 -> HalfBridgeMMC_Agt_Discrete/1(N)
  connections:
  1/RConn1 -- HalfBridgeMMC_Agt_Discrete/LConn1
  2/RConn1 -- HalfBridgeMMC_Agt_Discrete/LConn2

== system clearing_faulted_segment_travelling_Wave/MMC Converter1/Half-Bridge MMC Ap2 ==
  g : Inport
  HalfBridgeMMC_Agt_Discrete : Subsystem  mask{n=n, C=C, Vc_Initial=Vc_Initial, Ron_Diode=1e-3, Rs_Diode=1e6, Cs_Diode=inf, Vf_Diode=0}
      mask prompts: n "Number of bridges:"; C "Capacitor value (F):"; Vc_Initial "Initial capacitor voltage (V):"; Ron_Diode "Diode on-state resistance (Ohms)"; Rs_Diode "Diode snubber resistance (Ohms)"; Cs_Diode "Diode snubber capacitance (F)"; Vf_Diode "Diode forward voltage (V)"
  1 : PMIOPort  Side=Left
  2 : PMIOPort  Port=2  Side=Left
  Vc : Outport
  wires:
  g/1 -> HalfBridgeMMC_Agt_Discrete/1(N)
  HalfBridgeMMC_Agt_Discrete/1(Vc) -> Vc/1
  connections:
  2/RConn1 -- HalfBridgeMMC_Agt_Discrete/LConn2
  1/RConn1 -- HalfBridgeMMC_Agt_Discrete/LConn1

== system clearing_faulted_segment_travelling_Wave/MMC Converter1/Half-Bridge MMC Ap3 ==
  g : Inport
  HalfBridgeMMC_Agt_Discrete : Subsystem  mask{n=n, C=C, Vc_Initial=Vc_Initial, Ron_Diode=1e-3, Rs_Diode=1e6, Cs_Diode=inf, Vf_Diode=0}
      mask prompts: n "Number of bridges:"; C "Capacitor value (F):"; Vc_Initial "Initial capacitor voltage (V):"; Ron_Diode "Diode on-state resistance (Ohms)"; Rs_Diode "Diode snubber resistance (Ohms)"; Cs_Diode "Diode snubber capacitance (F)"; Vf_Diode "Diode forward voltage (V)"
  1 : PMIOPort  Side=Left
  2 : PMIOPort  Port=2  Side=Left
  Vc : Outport
  wires:
  g/1 -> HalfBridgeMMC_Agt_Discrete/1(N)
  HalfBridgeMMC_Agt_Discrete/1(Vc) -> Vc/1
  connections:
  2/RConn1 -- HalfBridgeMMC_Agt_Discrete/LConn2
  1/RConn1 -- HalfBridgeMMC_Agt_Discrete/LConn1

== system clearing_faulted_segment_travelling_Wave/MMC Converter1/Half-Bridge MMC Ap4 ==
  g : Inport
  HalfBridgeMMC_Agt_Discrete : Subsystem  mask{n=n, C=C, Vc_Initial=Vc_Initial, Ron_Diode=1e-3, Rs_Diode=1e6, Cs_Diode=inf, Vf_Diode=0}
      mask prompts: n "Number of bridges:"; C "Capacitor value (F):"; Vc_Initial "Initial capacitor voltage (V):"; Ron_Diode "Diode on-state resistance (Ohms)"; Rs_Diode "Diode snubber resistance (Ohms)"; Cs_Diode "Diode snubber capacitance (F)"; Vf_Diode "Diode forward voltage (V)"
  1 : PMIOPort  Side=Left
  2 : PMIOPort  Port=2  Side=Left
  Vc : Outport
  wires:
  HalfBridgeMMC_Agt_Discrete/1(Vc) -> Vc/1
  g/1 -> HalfBridgeMMC_Agt_Discrete/1(N)
  connections:
  1/RConn1 -- HalfBridgeMMC_Agt_Discrete/LConn1
  2/RConn1 -- HalfBridgeMMC_Agt_Discrete/LConn2

== system clearing_faulted_segment_travelling_Wave/MMC Converter1/Half-Bridge MMC Ap5 ==
  g : Inport
  HalfBridgeMMC_Agt_Discrete : Subsystem  mask{n=n, C=C, Vc_Initial=Vc_Initial, Ron_Diode=1e-3, Rs_Diode=1e6, Cs_Diode=inf, Vf_Diode=0}
      mask prompts: n "Number of bridges:"; C "Capacitor value (F):"; Vc_Initial "Initial capacitor voltage (V):"; Ron_Diode "Diode on-state resistance (Ohms)"; Rs_Diode "Diode snubber resistance (Ohms)"; Cs_Diode "Diode snubber capacitance (F)"; Vf_Diode "Diode forward voltage (V)"
  1 : PMIOPort  Side=Left
  2 : PMIOPort  Port=2  Side=Left
  Vc : Outport
  wires:
  g/1 -> HalfBridgeMMC_Agt_Discrete/1(N)
  HalfBridgeMMC_Agt_Discrete/1(Vc) -> Vc/1
  connections:
  2/RConn1 -- HalfBridgeMMC_Agt_Discrete/LConn2
  1/RConn1 -- HalfBridgeMMC_Agt_Discrete/LConn1

== system clearing_faulted_segment_travelling_Wave/MMC Converter2/Half-Bridge MMC Ap ==
  g : Inport
  HalfBridgeMMC_Agt_Discrete : Subsystem  mask{n=n, C=C, Vc_Initial=Vc_Initial, Ron_Diode=1e-3, Rs_Diode=1e6, Cs_Diode=inf, Vf_Diode=0}
      mask prompts: n "Number of bridges:"; C "Capacitor value (F):"; Vc_Initial "Initial capacitor voltage (V):"; Ron_Diode "Diode on-state resistance (Ohms)"; Rs_Diode "Diode snubber resistance (Ohms)"; Cs_Diode "Diode snubber capacitance (F)"; Vf_Diode "Diode forward voltage (V)"
  1 : PMIOPort  Side=Left
  2 : PMIOPort  Port=2  Side=Left
  Vc : Outport
  wires:
  HalfBridgeMMC_Agt_Discrete/1(Vc) -> Vc/1
  g/1 -> HalfBridgeMMC_Agt_Discrete/1(N)
  connections:
  1/RConn1 -- HalfBridgeMMC_Agt_Discrete/LConn1
  2/RConn1 -- HalfBridgeMMC_Agt_Discrete/LConn2

== system clearing_faulted_segment_travelling_Wave/MMC Converter2/Half-Bridge MMC Ap1 ==
  g : Inport
  HalfBridgeMMC_Agt_Discrete : Subsystem  mask{n=n, C=C, Vc_Initial=Vc_Initial, Ron_Diode=1e-3, Rs_Diode=1e6, Cs_Diode=inf, Vf_Diode=0}
      mask prompts: n "Number of bridges:"; C "Capacitor value (F):"; Vc_Initial "Initial capacitor voltage (V):"; Ron_Diode "Diode on-state resistance (Ohms)"; Rs_Diode "Diode snubber resistance (Ohms)"; Cs_Diode "Diode snubber capacitance (F)"; Vf_Diode "Diode forward voltage (V)"
  1 : PMIOPort  Side=Left
  2 : PMIOPort  Port=2  Side=Left
  Vc : Outport
  wires:
  HalfBridgeMMC_Agt_Discrete/1(Vc) -> Vc/1
  g/1 -> HalfBridgeMMC_Agt_Discrete/1(N)
  connections:
  1/RConn1 -- HalfBridgeMMC_Agt_Discrete/LConn1
  2/RConn1 -- HalfBridgeMMC_Agt_Discrete/LConn2

== system clearing_faulted_segment_travelling_Wave/MMC Converter2/Half-Bridge MMC Ap2 ==
  g : Inport
  HalfBridgeMMC_Agt_Discrete : Subsystem  mask{n=n, C=C, Vc_Initial=Vc_Initial, Ron_Diode=1e-3, Rs_Diode=1e6, Cs_Diode=inf, Vf_Diode=0}
      mask prompts: n "Number of bridges:"; C "Capacitor value (F):"; Vc_Initial "Initial capacitor voltage (V):"; Ron_Diode "Diode on-state resistance (Ohms)"; Rs_Diode "Diode snubber resistance (Ohms)"; Cs_Diode "Diode snubber capacitance (F)"; Vf_Diode "Diode forward voltage (V)"
  1 : PMIOPort  Side=Left
  2 : PMIOPort  Port=2  Side=Left
  Vc : Outport
  wires:
  g/1 -> HalfBridgeMMC_Agt_Discrete/1(N)
  HalfBridgeMMC_Agt_Discrete/1(Vc) -> Vc/1
  connections:
  2/RConn1 -- HalfBridgeMMC_Agt_Discrete/LConn2
  1/RConn1 -- HalfBridgeMMC_Agt_Discrete/LConn1

== system clearing_faulted_segment_travelling_Wave/MMC Converter2/Half-Bridge MMC Ap3 ==
  g : Inport
  HalfBridgeMMC_Agt_Discrete : Subsystem  mask{n=n, C=C, Vc_Initial=Vc_Initial, Ron_Diode=1e-3, Rs_Diode=1e6, Cs_Diode=inf, Vf_Diode=0}
      mask prompts: n "Number of bridges:"; C "Capacitor value (F):"; Vc_Initial "Initial capacitor voltage (V):"; Ron_Diode "Diode on-state resistance (Ohms)"; Rs_Diode "Diode snubber resistance (Ohms)"; Cs_Diode "Diode snubber capacitance (F)"; Vf_Diode "Diode forward voltage (V)"
  1 : PMIOPort  Side=Left
  2 : PMIOPort  Port=2  Side=Left
  Vc : Outport
  wires:
  g/1 -> HalfBridgeMMC_Agt_Discrete/1(N)
  HalfBridgeMMC_Agt_Discrete/1(Vc) -> Vc/1
  connections:
  2/RConn1 -- HalfBridgeMMC_Agt_Discrete/LConn2
  1/RConn1 -- HalfBridgeMMC_Agt_Discrete/LConn1

== system clearing_faulted_segment_travelling_Wave/MMC Converter2/Half-Bridge MMC Ap4 ==
  g : Inport
  HalfBridgeMMC_Agt_Discrete : Subsystem  mask{n=n, C=C, Vc_Initial=Vc_Initial, Ron_Diode=1e-3, Rs_Diode=1e6, Cs_Diode=inf, Vf_Diode=0}
      mask prompts: n "Number of bridges:"; C "Capacitor value (F):"; Vc_Initial "Initial capacitor voltage (V):"; Ron_Diode "Diode on-state resistance (Ohms)"; Rs_Diode "Diode snubber resistance (Ohms)"; Cs_Diode "Diode snubber capacitance (F)"; Vf_Diode "Diode forward voltage (V)"
  1 : PMIOPort  Side=Left
  2 : PMIOPort  Port=2  Side=Left
  Vc : Outport
  wires:
  HalfBridgeMMC_Agt_Discrete/1(Vc) -> Vc/1
  g/1 -> HalfBridgeMMC_Agt_Discrete/1(N)
  connections:
  1/RConn1 -- HalfBridgeMMC_Agt_Discrete/LConn1
  2/RConn1 -- HalfBridgeMMC_Agt_Discrete/LConn2

== system clearing_faulted_segment_travelling_Wave/MMC Converter2/Half-Bridge MMC Ap5 ==
  g : Inport
  HalfBridgeMMC_Agt_Discrete : Subsystem  mask{n=n, C=C, Vc_Initial=Vc_Initial, Ron_Diode=1e-3, Rs_Diode=1e6, Cs_Diode=inf, Vf_Diode=0}
      mask prompts: n "Number of bridges:"; C "Capacitor value (F):"; Vc_Initial "Initial capacitor voltage (V):"; Ron_Diode "Diode on-state resistance (Ohms)"; Rs_Diode "Diode snubber resistance (Ohms)"; Cs_Diode "Diode snubber capacitance (F)"; Vf_Diode "Diode forward voltage (V)"
  1 : PMIOPort  Side=Left
  2 : PMIOPort  Port=2  Side=Left
  Vc : Outport
  wires:
  g/1 -> HalfBridgeMMC_Agt_Discrete/1(N)
  HalfBridgeMMC_Agt_Discrete/1(Vc) -> Vc/1
  connections:
  2/RConn1 -- HalfBridgeMMC_Agt_Discrete/LConn2
  1/RConn1 -- HalfBridgeMMC_Agt_Discrete/LConn1

== system clearing_faulted_segment_travelling_Wave/MMC Converter3/Half-Bridge MMC Ap ==
  g : Inport
  HalfBridgeMMC_Agt_Discrete : Subsystem  mask{n=n, C=C, Vc_Initial=Vc_Initial, Ron_Diode=1e-3, Rs_Diode=1e6, Cs_Diode=inf, Vf_Diode=0}
      mask prompts: n "Number of bridges:"; C "Capacitor value (F):"; Vc_Initial "Initial capacitor voltage (V):"; Ron_Diode "Diode on-state resistance (Ohms)"; Rs_Diode "Diode snubber resistance (Ohms)"; Cs_Diode "Diode snubber capacitance (F)"; Vf_Diode "Diode forward voltage (V)"
  1 : PMIOPort  Side=Left
  2 : PMIOPort  Port=2  Side=Left
  Vc : Outport
  wires:
  HalfBridgeMMC_Agt_Discrete/1(Vc) -> Vc/1
  g/1 -> HalfBridgeMMC_Agt_Discrete/1(N)
  connections:
  1/RConn1 -- HalfBridgeMMC_Agt_Discrete/LConn1
  2/RConn1 -- HalfBridgeMMC_Agt_Discrete/LConn2

== system clearing_faulted_segment_travelling_Wave/MMC Converter3/Half-Bridge MMC Ap1 ==
  g : Inport
  HalfBridgeMMC_Agt_Discrete : Subsystem  mask{n=n, C=C, Vc_Initial=Vc_Initial, Ron_Diode=1e-3, Rs_Diode=1e6, Cs_Diode=inf, Vf_Diode=0}
      mask prompts: n "Number of bridges:"; C "Capacitor value (F):"; Vc_Initial "Initial capacitor voltage (V):"; Ron_Diode "Diode on-state resistance (Ohms)"; Rs_Diode "Diode snubber resistance (Ohms)"; Cs_Diode "Diode snubber capacitance (F)"; Vf_Diode "Diode forward voltage (V)"
  1 : PMIOPort  Side=Left
  2 : PMIOPort  Port=2  Side=Left
  Vc : Outport
  wires:
  HalfBridgeMMC_Agt_Discrete/1(Vc) -> Vc/1
  g/1 -> HalfBridgeMMC_Agt_Discrete/1(N)
  connections:
  1/RConn1 -- HalfBridgeMMC_Agt_Discrete/LConn1
  2/RConn1 -- HalfBridgeMMC_Agt_Discrete/LConn2
